simulink model "machineOne"  (R2021a)
settings: Solver=VariableStepAuto  StartTime=0.0  StopTime=10.0  RelTol=1e-3
settings Model: Creator=iumrikhin  LastModifiedBy=iumrikhin

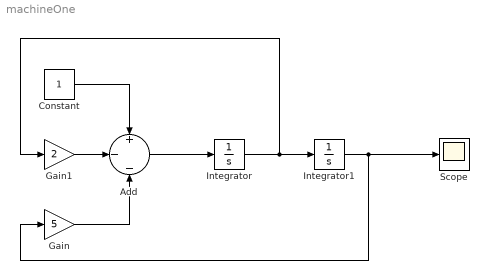
== system machineOne ==
  Add : Sum  Inputs=+|-|-
  Constant : Constant
  Gain : Gain  Gain=5
  Gain1 : Gain  Gain=2
  Integrator : Integrator
  Integrator1 : Integrator
  Scope : Scope
  wires:
  Gain1/1 -> Add/2
  Gain/1 -> Add/3
  Constant/1 -> Add/1
  Add/1 -> Integrator/1
  Integrator/1 -> Gain1/1, Integrator1/1
  Integrator1/1 -> Scope/1, Gain/1
